simulink model "Throttle_Velocity_Dynamics_Ex3"  (R2023a)
settings: Solver=VariableStepAuto  StartTime=0.0  StopTime=20.0  RelTol=1e-3
undefined symbols (not defined in the file): a, b, bm, d, gamma1, gamma2, gamma3
settings Model: Creator=geokr  LastModifiedBy=geokr

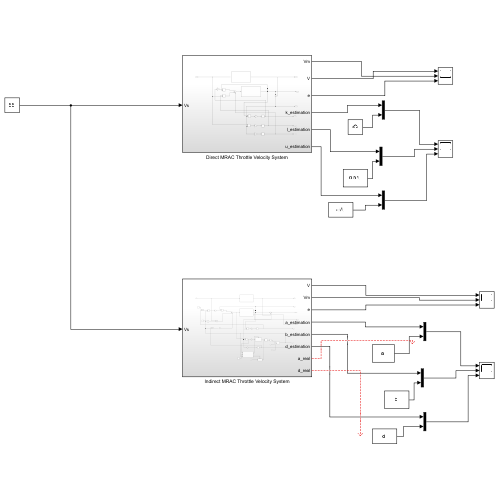
[thumbnail: Simulink's stored preview of the top-level diagram]
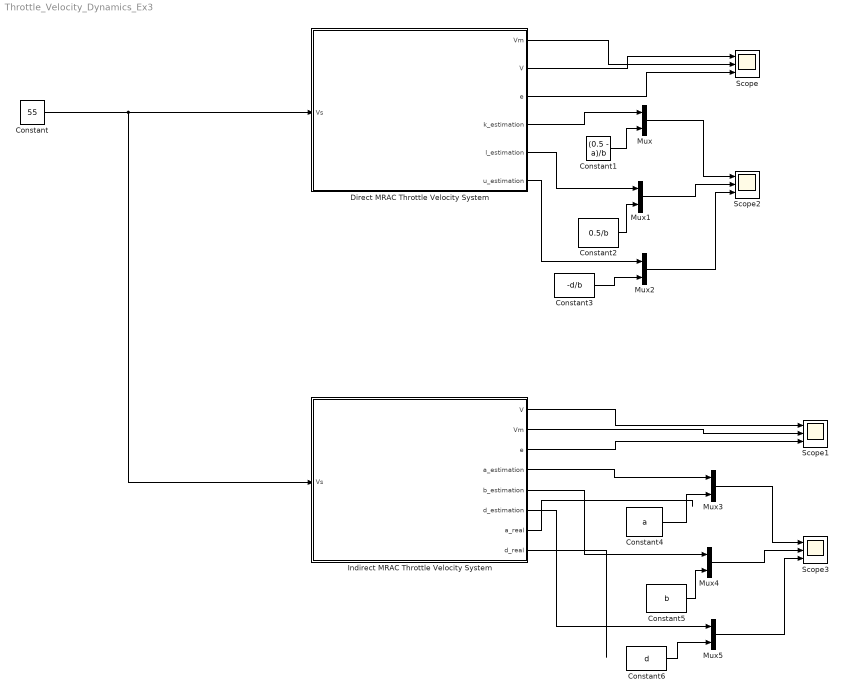
== system Throttle_Velocity_Dynamics_Ex3 ==
  Constant : Constant  Value=55
  Constant1 : Constant  Value=(0.5 - a)/b
  Constant2 : Constant  Value=0.5/b
  Constant3 : Constant  Value=-d/b
  Constant4 : Constant  Value=a
  Constant5 : Constant  Value=b
  Constant6 : Constant  Value=d
  Direct MRAC Throttle Velocity System : Subsystem
  Indirect MRAC Throttle Velocity System : Subsystem
  Mux{,1..5} (6 alike) : Mux  Inputs=2
  Scope{,1..3} (4 alike) : Scope  NumInputPorts=3
  wires:
  Direct MRAC Throttle Velocity System/4(k_estimation) -> Mux/1
  Indirect MRAC Throttle Velocity System/5(b_estimation) -> Mux4/1
  Indirect MRAC Throttle Velocity System/4(a_estimation) -> Mux3/1
  Mux2/1 -> Scope2/3
  Mux/1 -> Scope2/1
  Direct MRAC Throttle Velocity System/2(V) -> Scope/1
  Direct MRAC Throttle Velocity System/3(e) -> Scope/3
  Direct MRAC Throttle Velocity System/6(u_estimation) -> Mux2/1
  Constant3/1 -> Mux2/2
  Direct MRAC Throttle Velocity System/5(l_estimation) -> Mux1/1
  Constant1/1 -> Mux/2
  Constant2/1 -> Mux1/2
  Indirect MRAC Throttle Velocity System/3(e) -> Scope1/3
  Mux4/1 -> Scope3/2
  Constant5/1 -> Mux4/2
  Mux3/1 -> Scope3/1
  Mux5/1 -> Scope3/3
  Indirect MRAC Throttle Velocity System/6(d_estimation) -> Mux5/1
  Mux1/1 -> Scope2/2
  Direct MRAC Throttle Velocity System/1(Vm) -> Scope/2
  Constant/1 -> Direct MRAC Throttle Velocity System/1(Vs), Indirect MRAC Throttle Velocity System/1(Vs)
  Indirect MRAC Throttle Velocity System/1(V) -> Scope1/1
  Indirect MRAC Throttle Velocity System/2(Vm) -> Scope1/2
  Constant4/1 -> Mux3/2
  Indirect MRAC Throttle Velocity System/7(a_real) -> ?
  Indirect MRAC Throttle Velocity System/8(d_real) -> ?
  Constant6/1 -> Mux5/2

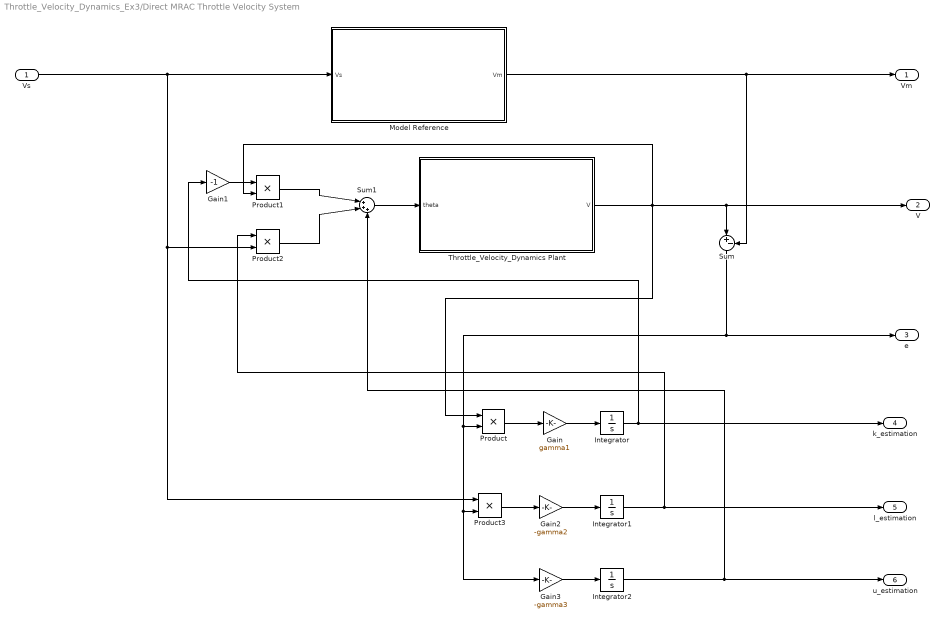
== system Throttle_Velocity_Dynamics_Ex3/Direct MRAC Throttle Velocity System ==
  Vs : Inport
  Gain : Gain  Gain=gamma1
  Gain1 : Gain  Gain=-1
  Gain2 : Gain  Gain=-gamma2
  Gain3 : Gain  Gain=-gamma3
  Integrator : Integrator
  Integrator1 : Integrator
  Integrator2 : Integrator
  Model Reference : Subsystem
  Product{,1..3} (4 alike) : Product
  Sum : Sum  Inputs=|+-
  Sum1 : Sum  Inputs=|+++
  Throttle_Velocity_Dynamics Plant : Subsystem
  Vm : Outport
  V : Outport  Port=2
  e : Outport  Port=3
  k_estimation : Outport  Port=4
  l_estimation : Outport  Port=5
  u_estimation : Outport  Port=6
  wires:
  Model Reference/1(Vm) -> Vm/1, Sum/2
  Product1/1 -> Sum1/1
  Vs/1 -> Model Reference/1(Vs), Product3/1, Product2/2
  Product2/1 -> Sum1/2
  Integrator/1 -> k_estimation/1, Gain1/1
  Sum/1 -> e/1, Product3/2, Gain3/1, Product/2
  Gain3/1 -> Integrator2/1
  Throttle_Velocity_Dynamics Plant/1(V) -> Product1/2, Product/1, V/1, Sum/1
  Sum1/1 -> Throttle_Velocity_Dynamics Plant/1(theta)
  Gain/1 -> Integrator/1
  Integrator1/1 -> l_estimation/1, Product2/1
  Gain1/1 -> Product1/1
  Product/1 -> Gain/1
  Product3/1 -> Gain2/1
  Integrator2/1 -> u_estimation/1, Sum1/3
  Gain2/1 -> Integrator1/1

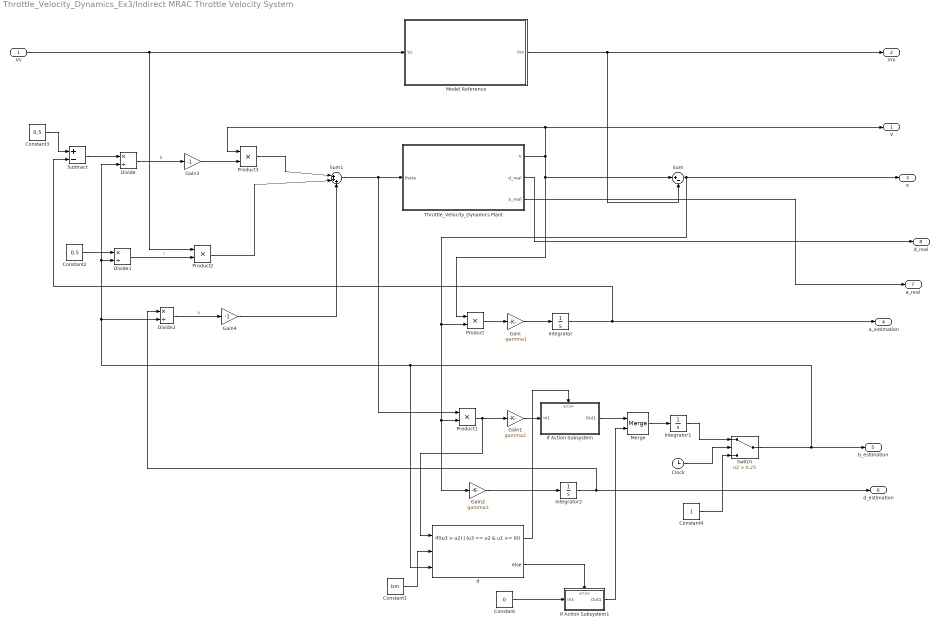
== system Throttle_Velocity_Dynamics_Ex3/Indirect MRAC Throttle Velocity System ==
  Vs : Inport
  Clock : Clock
  Constant : Constant  Value=0
  Constant1 : Constant  Value=bm
  Constant2 : Constant  Value=0.5
  Constant3 : Constant  Value=0.5
  Constant4 : Constant
  Divide : Product  Inputs=*/
  Divide1 : Product  Inputs=*/
  Divide2 : Product  Inputs=*/
  Gain : Gain  Gain=-gamma1
  Gain1 : Gain  Gain=gamma2
  Gain2 : Gain  Gain=gamma3
  Gain3 : Gain  Gain=-1
  Gain4 : Gain  Gain=-1
  If : If  NumInputs=3  IfExpression=(u3 > u2) | (u3 == u2 & u1 >= 0)
  If Action Subsystem : Subsystem  TreatAsAtomicUnit=on
  If Action Subsystem1 : Subsystem  TreatAsAtomicUnit=on
  Integrator : Integrator
  Integrator1 : Integrator
  Integrator2 : Integrator
  Merge : Merge
  Model Reference : Subsystem
  Product{,1..3} (4 alike) : Product
  Subtract : Sum  Inputs=+-
  Sum : Sum  Inputs=|+-
  Sum1 : Sum  Inputs=|+++
  Switch : Switch  Criteria=u2 > Threshold  Threshold=0.25  SaturateOnIntegerOverflow=off  InputSameDT=off
  Throttle_Velocity_Dynamics Plant : Subsystem
  V : Outport
  Vm : Outport  Port=2
  e : Outport  Port=3
  a_estimation : Outport  Port=4
  b_estimation : Outport  Port=5
  d_estimation : Outport  Port=6
  a_real : Outport  Port=7
  d_real : Outport  Port=8
  wires:
  Vs/1 -> Product2/1, Model Reference/1(Vs)
  Model Reference/1(Vm) -> Sum/2, Vm/1
  Throttle_Velocity_Dynamics Plant/1(V) -> Product/1, Sum/1, Product3/1, V/1
  Sum/1 -> Product/2, Product1/2, Gain2/1, e/1
  Gain/1 -> Integrator/1
  Product/1 -> Gain/1
  Integrator/1 -> Subtract/2, a_estimation/1
  Gain2/1 -> Integrator2/1
  Product1/1 -> If/1, Gain1/1
  Constant/1 -> If Action Subsystem1/1(In1)
  If/2 -> If Action Subsystem1/Action
  If/1 -> If Action Subsystem/Action
  Gain1/1 -> If Action Subsystem/1(In1)
  Merge/1 -> Integrator1/1
  If Action Subsystem/1(Out1) -> Merge/1
  If Action Subsystem1/1(Out1) -> Merge/2
  Integrator2/1 -> Divide2/1, d_estimation/1
  Sum1/1 -> Throttle_Velocity_Dynamics Plant/1(theta), Product1/1
  Constant1/1 -> If/2
  Divide/1 -> Gain3/1  "k"
  Divide1/1 -> Product2/2  "l"
  Divide2/1 -> Gain4/1  "u"
  Gain3/1 -> Product3/2
  Product3/1 -> Sum1/1
  Product2/1 -> Sum1/2
  Gain4/1 -> Sum1/3
  Constant2/1 -> Divide1/1
  Subtract/1 -> Divide/1
  Constant3/1 -> Subtract/1
  Clock/1 -> Switch/2
  Integrator1/1 -> Switch/1
  Constant4/1 -> Switch/3
  Switch/1 -> If/3, Divide2/2, Divide1/2, Divide/2, b_estimation/1
  Throttle_Velocity_Dynamics Plant/2(d_real) -> d_real/1
  Throttle_Velocity_Dynamics Plant/3(a_real) -> a_real/1

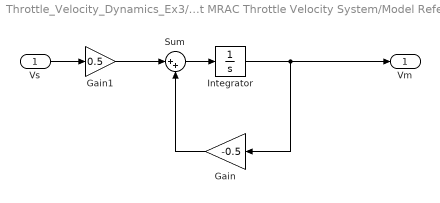
== system Throttle_Velocity_Dynamics_Ex3/Direct MRAC Throttle Velocity System/Model Reference ==
  Vs : Inport
  Gain : Gain  Gain=-0.5
  Gain1 : Gain  Gain=0.5
  Integrator : Integrator
  Sum : Sum  Inputs=|++
  Vm : Outport
  wires:
  Sum/1 -> Integrator/1
  Integrator/1 -> Gain/1, Vm/1
  Gain/1 -> Sum/2
  Vs/1 -> Gain1/1
  Gain1/1 -> Sum/1

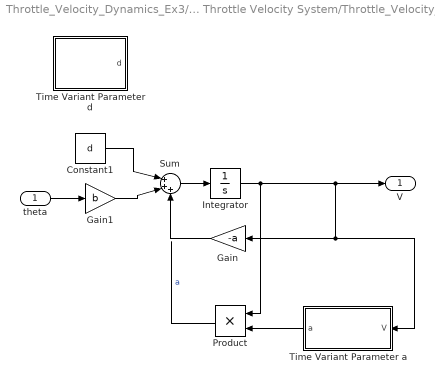
== system Throttle_Velocity_Dynamics_Ex3/Direct MRAC Throttle Velocity System/Throttle_Velocity_Dynamics Plant ==
  theta : Inport
  Constant1 : Constant  Value=d
  Gain : Gain  Gain=-a
  Gain1 : Gain  Gain=b
  Integrator : Integrator
  Product : Product
  Sum : Sum  Inputs=|+++
  Time Variant Parameter a : Subsystem
  Time Variant Parameter d : Subsystem
  V : Outport
  wires:
  Integrator/1 -> Time Variant Parameter a/1(V), Gain/1, V/1, Product/1
  Sum/1 -> Integrator/1
  theta/1 -> Gain1/1
  Gain1/1 -> Sum/2
  Time Variant Parameter a/1(a) -> Product/2
  Product/1 -> ?  "a"
  Gain/1 -> Sum/3
  Constant1/1 -> Sum/1

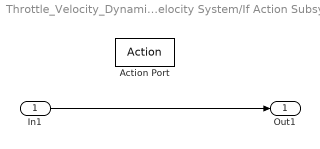
== system Throttle_Velocity_Dynamics_Ex3/Indirect MRAC Throttle Velocity System/If Action Subsystem ==
  In1 : Inport
  Action Port : ActionPort  ActionPortLabel=if((u3 > u2) | (u3 == u2 & u1 >= 0))
  Out1 : Outport
  wires:
  In1/1 -> Out1/1

== system Throttle_Velocity_Dynamics_Ex3/Indirect MRAC Throttle Velocity System/If Action Subsystem1 ==
  In1 : Inport
  Action Port : ActionPort  ActionPortLabel=else
  Out1 : Outport
  wires:
  In1/1 -> Out1/1

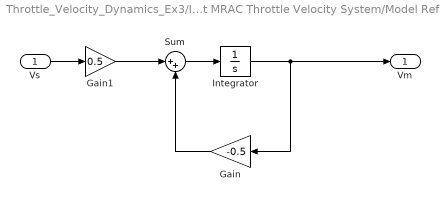
== system Throttle_Velocity_Dynamics_Ex3/Indirect MRAC Throttle Velocity System/Model Reference ==
  Vs : Inport
  Gain : Gain  Gain=-0.5
  Gain1 : Gain  Gain=0.5
  Integrator : Integrator
  Sum : Sum  Inputs=|++
  Vm : Outport
  wires:
  Sum/1 -> Integrator/1
  Integrator/1 -> Gain/1, Vm/1
  Gain/1 -> Sum/2
  Vs/1 -> Gain1/1
  Gain1/1 -> Sum/1

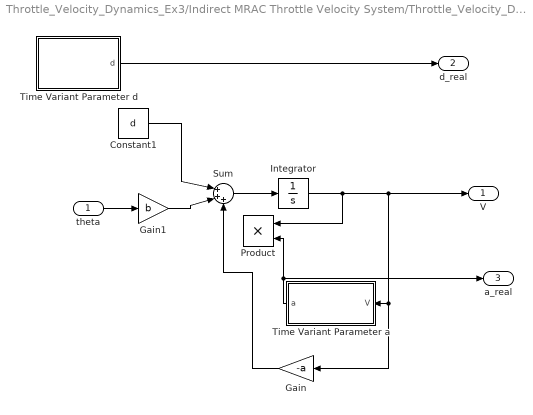
== system Throttle_Velocity_Dynamics_Ex3/Indirect MRAC Throttle Velocity System/Throttle_Velocity_Dynamics Plant ==
  theta : Inport
  Constant1 : Constant  Value=d
  Gain : Gain  Gain=-a
  Gain1 : Gain  Gain=b
  Integrator : Integrator
  Product : Product
  Sum : Sum  Inputs=|+++
  Time Variant Parameter a : Subsystem
  Time Variant Parameter d : Subsystem
  V : Outport
  d_real : Outport  Port=2
  a_real : Outport  Port=3
  wires:
  Integrator/1 -> Product/1, Time Variant Parameter a/1(V), Gain/1, V/1
  Sum/1 -> Integrator/1
  theta/1 -> Gain1/1
  Gain1/1 -> Sum/2
  Time Variant Parameter a/1(a) -> Product/2, a_real/1
  Constant1/1 -> Sum/1
  Gain/1 -> Sum/3
  Time Variant Parameter d/1(d) -> d_real/1

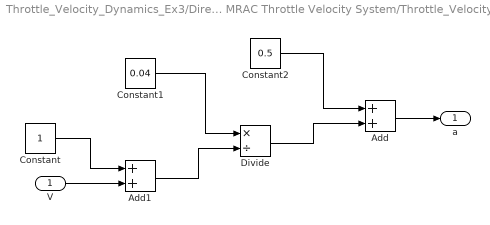
== system Throttle_Velocity_Dynamics_Ex3/Direct MRAC Throttle Velocity System/Throttle_Velocity_Dynamics Plant/Time Variant Parameter a ==
  V : Inport
  Add : Sum
  Add1 : Sum
  Constant : Constant
  Constant1 : Constant  Value=0.04
  Constant2 : Constant  Value=0.5
  Divide : Product  Inputs=*/
  a : Outport
  wires:
  Add/1 -> a/1
  Divide/1 -> Add/2
  Add1/1 -> Divide/2
  V/1 -> Add1/2
  Constant/1 -> Add1/1
  Constant1/1 -> Divide/1
  Constant2/1 -> Add/1

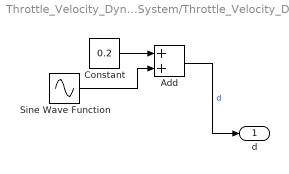
== system Throttle_Velocity_Dynamics_Ex3/Direct MRAC Throttle Velocity System/Throttle_Velocity_Dynamics Plant/Time Variant Parameter d ==
  Add : Sum
  Constant : Constant  Value=0.2
  Sine Wave Function : Sin  Frequency=0.02  SampleTime=0
  d : Outport
  wires:
  Sine Wave Function/1 -> Add/2
  Constant/1 -> Add/1
  Add/1 -> d/1  "d"

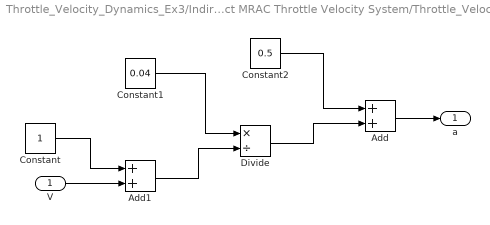
== system Throttle_Velocity_Dynamics_Ex3/Indirect MRAC Throttle Velocity System/Throttle_Velocity_Dynamics Plant/Time Variant Parameter a ==
  V : Inport
  Add : Sum
  Add1 : Sum
  Constant : Constant
  Constant1 : Constant  Value=0.04
  Constant2 : Constant  Value=0.5
  Divide : Product  Inputs=*/
  a : Outport
  wires:
  Add/1 -> a/1
  Divide/1 -> Add/2
  Add1/1 -> Divide/2
  V/1 -> Add1/2
  Constant/1 -> Add1/1
  Constant1/1 -> Divide/1
  Constant2/1 -> Add/1

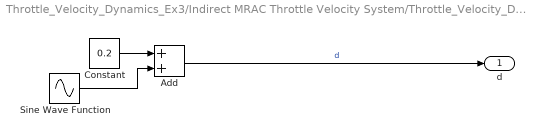
== system Throttle_Velocity_Dynamics_Ex3/Indirect MRAC Throttle Velocity System/Throttle_Velocity_Dynamics Plant/Time Variant Parameter d ==
  Add : Sum
  Constant : Constant  Value=0.2
  Sine Wave Function : Sin  Frequency=0.02  SampleTime=0
  d : Outport
  wires:
  Constant/1 -> Add/1
  Add/1 -> d/1  "d"
  Sine Wave Function/1 -> Add/2
